simulink model "AllinOne"  (R2017a)
settings: Solver=ode3  StartTime=0.0  StopTime=Inf  RelTol=1e-3  EnableMultiTasking=on
StopFcn:
  | CoffeeMachineIOSupport('closefig');
libraries: pil_lib x1
settings Model: DataDictionary=Struct.sldd  NumberOfSteps=100  ParamWorkspaceSource=ReferencedWorkspace  Creator=89YY  LastModifiedBy=dell1
settings DataIOCC: LimitDataPoints=on  SaveFormat=Array
settings OptimizationCC: UseFloatMulNetSlope=on  PassReuseOutputArgsAs=Individual arguments  ZeroExternalMemoryAtStartup=off  ZeroInternalMemoryAtStartup=off  NoFixptDivByZeroProtection=on  EfficientFloat2IntCast=on  LifeSpan=1  MaxStackSize=64
settings DebuggingCC: SaveWithParameterizedLinksMsg=none  UnderspecifiedInitializationDetection=Classic  MergeDetectMultiDrivingBlocksExec=none  SFUnexpectedBacktrackingDiag=warning  SFNoUnconditionalDefaultTransitionDiag=warning  SFExecutionAtInitializationDiag=none
settings HardwareCC: ProdBitPerPointer=32  ProdBitPerSizeT=32  ProdBitPerPtrDiffT=32  ProdLargestAtomicInteger=Long  ProdLargestAtomicFloat=Double  ProdWordSize=32  ProdHWDeviceType=ARM Compatible->ARM Cortex  TargetBitPerPointer=64  TargetBitPerSizeT=64  TargetBitPerPtrDiffT=64  TargetLongLongMode=on  TargetIntDivRoundTo=Zero  TargetEndianess=LittleEndian  TargetWordSize=64  TargetHWDeviceType=MATLAB Host  ProdEqTarget=off
settings ModelReferenceCC: PropagateSignalLabelsOutOfModel=off
settings SFSimCC: MATLABDynamicMemAlloc=off
settings RTWCC: SystemTargetFile=ert.tlc  HardwareBoard=ARM Cortex-M3 (QEMU)  TLCOptions=-aInlineSetEventsForThisBaseRateFcn=TLC_FALSE -aSuppressMultiTaskScheduler=TLC_FALSE -aRateBasedStepFcn=1  TemplateMakefile=ert_default_tmf  Description=Embedded Coder  GenerateReport=on  Toolchain=GNU Tools for ARM Embedded Processors  IncludeHyperlinkInReport=on  LaunchReport=on  CreateSILPILBlock=PIL  GenerateTraceInfo=on  GenerateTraceReport=on  GenerateTraceReportSl=on  GenerateTraceReportSf=on  GenerateTraceReportEml=on  GenerateCodeMetricsReport=on
settings CodeAppCC: ForceParamTrailComments=on  IgnoreCustomStorageClasses=off  SimulinkDataObjDesc=on  CustomSymbolStrGlobalVar=rt$N$M  CustomSymbolStrType=$N$M  CustomSymbolStrFcn=$N$M$F  CustomSymbolStrMacro=$N$M  InsertBlockDesc=on
settings ERTTargetCC: MultiwordLength=2048  IncludeMdlTerminateFcn=off  CombineSignalStateStructs=on  SupportNonFinite=off  ERTFilePackagingFormat=CompactWithDataFile  ConvertIfToSwitch=off  SuppressUnreachableDefaultCases=off
settings ConfigComp: CovMetricSettings=dw  CovHtmlReporting=on  CovSaveCumulativeToWorkspaceVar=on  CovSaveSingleToWorkspaceVar=on  CovExternalEMLEnable=off  CovSFcnEnable=off

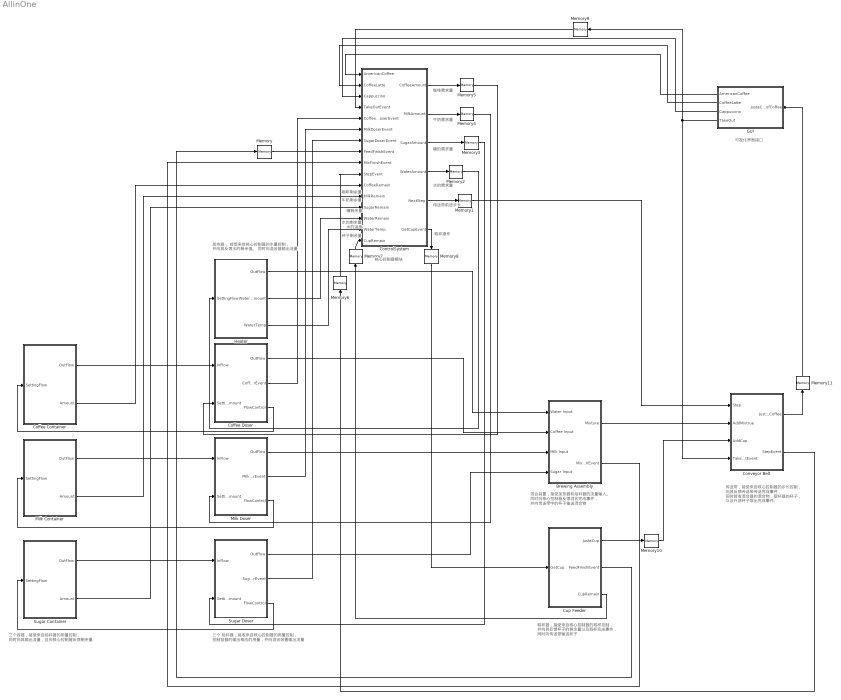
== system AllinOne ==
  note: 水的需求量
  note: 可视化界面接口
  note: 加热器， 接受来自核心控制器的水量控制，
      | 并向其反馈水的剩余值。
      | 同时向混合器输出流量
  note: 传送带，接受来自核心控制器的步长控制，
      | 向其反馈传送带传送完成事件，
      | 同时接收混合器的混合物，取杯器的杯子，
      | 以及外部杯子取出完成事件。
  note: 混合装置，接受加热器和给料器的流量输入。
      | 同时向核心控制器反馈混合完成事件，
      | 并向传送带中的杯子输送混合物
  note: 取杯器，接受来自核心控制器的取杯控制，
      | 并向其反馈杯子的剩余量以及取杯完成事件，
      | 同时向传送带输送杯子
  note: 三个 给料器，接收来自核心控制器的用量控制，
      | 控制容器的输出相应的用量，并向混合装置输出流量
  note: 三个容器，接受来自给料器的用量控制，
      | 同时向其输出流量，且向核心控制器反馈剩余量
  note: 取杯操作
  note: 传送带前进步长
  note: 糖的需求量
  note: 牛奶需求量
  note: 咖啡需求量
  note: 杯子剩余量
  note: 水的温度
  note: 水的剩余量
  note: 糖剩余量
  note: 牛奶剩余量
  note: 咖啡剩余量
  note: 核心控制器模块
  Brewing Assembly : Subsystem
  Coffee Container : Subsystem
  Coffee Doser : Subsystem
  ControlSystem : Subsystem  DialogController=pil_create_dialog  LoadFcn=|
      | try
      |    if ~strcmp(rtw.pil.getPILVersion, '6.12 (R2017a)_12')
      |       set_param(gcb, 'DialogController', '');
      |       set_param(gcb, 'DialogControllerArgs', '');
      |    end
      | catch e
      |       set_param(gcb, 'DialogController', '');
      |       set_param(gcb, 'DialogControllerArgs', '');
      | end
      mask help: PIL:pil:XILBlockMaskDesc
      mask Display: disp('PIL');
  Conveyor Belt : Subsystem
  Cup Feeder : Subsystem
  GUI : Subsystem
  Heater : Subsystem
  Memory{,1..11} (12 alike) : Memory
  Milk Container : Subsystem
  Milk Doser : Subsystem
  Sugar Container : Subsystem
  Sugar Doser : Subsystem
  wires:
  Milk Container/1(OutFlow) -> Milk Doser/1(InFlow)
  Milk Doser/3(FlowControl) -> Milk Container/1(SettingFlow)
  Coffee Container/1(OutFlow) -> Coffee Doser/1(InFlow)
  Coffee Doser/3(FlowControl) -> Coffee Container/1(SettingFlow)
  Sugar Container/1(OutFlow) -> Sugar Doser/1(InFlow)
  Sugar Doser/3(FlowControl) -> Sugar Container/1(SettingFlow)
  Coffee Doser/1(OutFlow) -> Brewing Assembly/2(Coffee Input)
  Milk Doser/1(OutFlow) -> Brewing Assembly/3(Milk Input)
  Sugar Doser/1(OutFlow) -> Brewing Assembly/4(Sugar Input)
  Brewing Assembly/1(Mixture) -> Conveyor Belt/2(AddMixtrue)
  Cup Feeder/1(JustaCup) -> Memory10/1
  Heater/1(OutFlow) -> Brewing Assembly/1(Water Input)
  GUI/4(TakeOut) -> Memory9/1, Conveyor Belt/4(TakeOutEvent)
  Conveyor Belt/1(JustaCupofCoffee) -> Memory11/1
  GUI/3(Cappuccino) -> ControlSystem/3(Cappuccino)
  GUI/2(CoffeeLatte) -> ControlSystem/2(CoffeeLatte)
  GUI/1(AmericanCoffee) -> ControlSystem/1(AmericanCoffee)
  Coffee Doser/2(CoffeeDoserEvent) -> ControlSystem/5(CoffeeDoserEvent)
  Milk Doser/2(MilkDoserEvent) -> ControlSystem/6(MilkDoserEvent)
  Sugar Doser/2(SugarDoserEvent) -> ControlSystem/7(SugarDoserEvent)
  Coffee Container/2(Amount) -> ControlSystem/11(CoffeeRemain)
  Milk Container/2(Amount) -> ControlSystem/12(MilkRemain)
  Sugar Container/2(Amount) -> ControlSystem/13(SugarRemain)
  Heater/2(WaterAmount) -> ControlSystem/14(WaterRemain)
  Heater/3(WaterTemp) -> ControlSystem/15(WaterTemp)
  Cup Feeder/3(CupRemain) -> Memory7/1
  Brewing Assembly/2(MixFinishEvent) -> ControlSystem/9(MixFinishEvent)
  Cup Feeder/2(FeedFinishEvent) -> Memory/1
  Conveyor Belt/2(StepEvent) -> Memory6/1
  ControlSystem/1(CoffeeAmount) -> Memory5/1
  ControlSystem/2(MilkAmount) -> Memory4/1
  ControlSystem/3(SugarAmount) -> Memory3/1
  ControlSystem/5(NextStep) -> Memory1/1
  ControlSystem/4(WaterAmount) -> Memory2/1
  Memory5/1 -> Coffee Doser/2(SettingAmount)
  Memory4/1 -> Milk Doser/2(SettingAmount)
  Memory3/1 -> Sugar Doser/2(SettingAmount)
  Memory2/1 -> Heater/1(SettingFlow)
  Memory1/1 -> Conveyor Belt/1(Step)
  ControlSystem/6(GetCupEvent) -> Memory8/1
  Memory/1 -> ControlSystem/8(FeedFinishEvent)
  Memory6/1 -> ControlSystem/10(StepEvent)
  Memory7/1 -> ControlSystem/16(CupRemain)
  Memory8/1 -> Cup Feeder/1(GetCup)
  Memory9/1 -> ControlSystem/4(TakeOutEvent)
  Memory10/1 -> Conveyor Belt/3(AddCup)
  Memory11/1 -> GUI/1(JustaCupofCoffee)

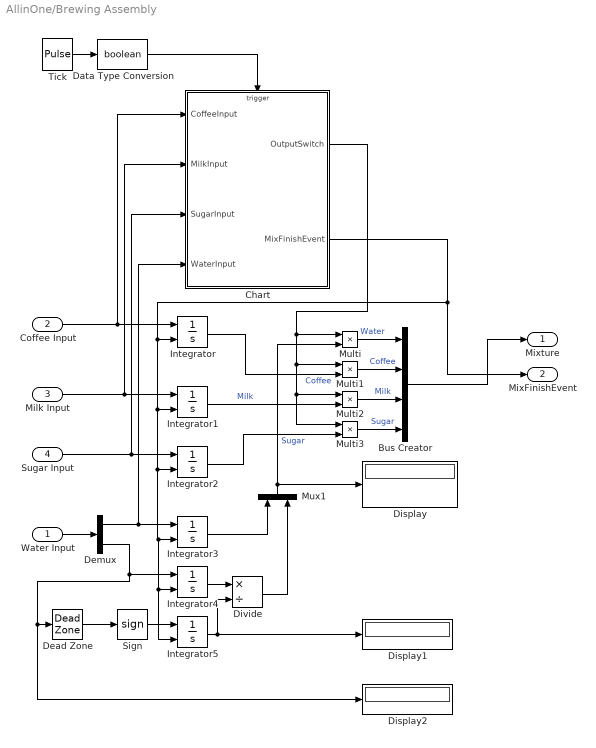
== system AllinOne/Brewing Assembly ==
  Water Input : Inport
  Coffee Input : Inport  Port=2
  Milk Input : Inport  Port=3
  Sugar Input : Inport  Port=4
  Bus Creator : BusCreator  Inputs=4  OutDataTypeStr=Bus: Mixtrue
  Chart : Stateflow chart  TreatAsAtomicUnit=on
  Data Type Conversion : DataTypeConversion  OutDataTypeStr=boolean
  Dead Zone : DeadZone  LowerValue=-1e-5  UpperValue=1e-5  SaturateOnIntegerOverflow=on
  Demux : Demux  Outputs=2
  Display : Display
  Display1 : Display
  Display2 : Display
  Divide : Product  Inputs=*/
  Integrator{,1..5} (6 alike) : Integrator  ExternalReset=rising
  Multi{,1..3} (4 alike) : Product  Inputs=**
  Mux1 : Mux  Inputs=2
  Sign : Signum
  Tick : DiscretePulseGenerator  PulseType=Time based  Period=0.01  PulseWidth=50
  Mixture : Outport  OutDataTypeStr=Bus: Mixtrue
  MixFinishEvent : Outport  Port=2
  wires:
  Tick/1 -> Data Type Conversion/1
  Data Type Conversion/1 -> Chart/Trigger
  Sugar Input/1 -> Integrator2/1, Chart/3(SugarInput)
  Demux/1 -> Chart/4(WaterInput), Integrator3/1
  Milk Input/1 -> Integrator1/1, Chart/2(MilkInput)
  Coffee Input/1 -> Integrator/1, Chart/1(CoffeeInput)
  Chart/2(MixFinishEvent) -> MixFinishEvent/1, Integrator5/2, Integrator4/2, Integrator3/2, Integrator2/2, Integrator1/2, Integrator/2
  Multi1/1 -> Bus Creator/2  "Coffee"
  Mux1/1 -> Multi/2, Display/1
  Multi2/1 -> Bus Creator/3  "Milk"
  Multi3/1 -> Bus Creator/4  "Sugar"
  Bus Creator/1 -> Mixture/1
  Chart/1(OutputSwitch) -> Multi3/1, Multi2/1, Multi1/1, Multi/1
  Water Input/1 -> Demux/1
  Integrator3/1 -> Mux1/1
  Sign/1 -> Integrator5/1
  Demux/2 -> Display2/1, Dead Zone/1, Integrator4/1
  Integrator4/1 -> Divide/1
  Integrator5/1 -> Display1/1, Divide/2
  Divide/1 -> Mux1/2
  Multi/1 -> Bus Creator/1  "Water"
  Integrator/1 -> Multi1/2  "Coffee"
  Integrator1/1 -> Multi2/2  "Milk"
  Integrator2/1 -> Multi3/2  "Sugar"
  Dead Zone/1 -> Sign/1

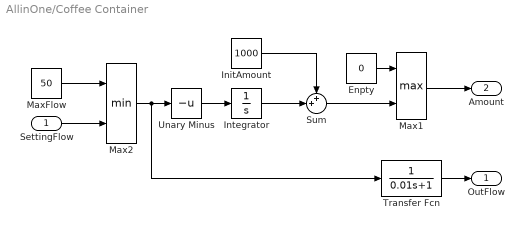
== system AllinOne/Coffee Container ==
  SettingFlow : Inport
  Enpty : Constant  Value=0
  InitAmount : Constant  Value=1000
  Integrator : Integrator
  Max1 : MinMax  Function=max  Inputs=2
  Max2 : MinMax  Inputs=2  OutMin=[0]
  MaxFlow : Constant  Value=50
  Sum : Sum  Inputs=++|
  Transfer Fcn : TransferFcn  Denominator=[0.01 1]
  Unary Minus : UnaryMinus
  OutFlow : Outport
  Amount : Outport  Port=2
  wires:
  Unary Minus/1 -> Integrator/1
  Integrator/1 -> Sum/2
  SettingFlow/1 -> Max2/2
  InitAmount/1 -> Sum/1
  Max2/1 -> Transfer Fcn/1, Unary Minus/1
  MaxFlow/1 -> Max2/1
  Max1/1 -> Amount/1
  Sum/1 -> Max1/2
  Enpty/1 -> Max1/1
  Transfer Fcn/1 -> OutFlow/1

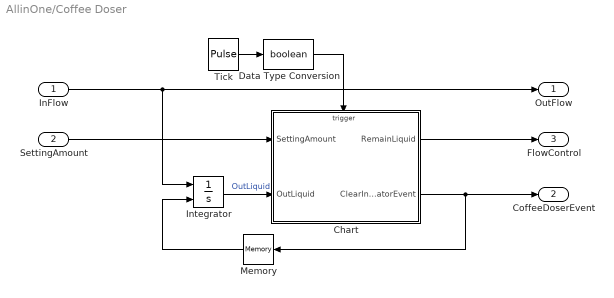
== system AllinOne/Coffee Doser ==
  InFlow : Inport
  SettingAmount : Inport  Port=2
  Chart : Stateflow chart  RequirementInfo={} %GIDa_ffed56c2_cd34_4288_8248_c4489554cc95  TreatAsAtomicUnit=on
  Data Type Conversion : DataTypeConversion  OutDataTypeStr=boolean
  Integrator : Integrator  ExternalReset=rising
  Memory : Memory
  Tick : DiscretePulseGenerator  PulseType=Time based  Period=0.01  PulseWidth=50
  OutFlow : Outport
  CoffeeDoserEvent : Outport  Port=2
  FlowControl : Outport  Port=3
  wires:
  SettingAmount/1 -> Chart/1(SettingAmount)
  Chart/1(RemainLiquid) -> FlowControl/1
  InFlow/1 -> OutFlow/1, Integrator/1
  Chart/2(ClearIntegratorEvent) -> Memory/1, CoffeeDoserEvent/1
  Integrator/1 -> Chart/2(OutLiquid)  "OutLiquid"
  Tick/1 -> Data Type Conversion/1
  Data Type Conversion/1 -> Chart/Trigger
  Memory/1 -> Integrator/2

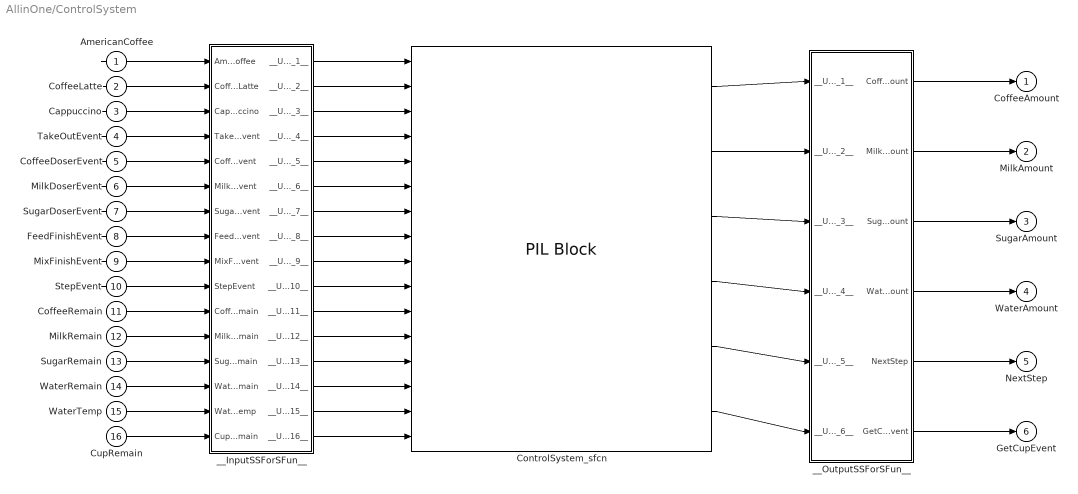
== system AllinOne/ControlSystem ==
  AmericanCoffee : Inport
  CoffeeLatte : Inport  Port=2
  Cappuccino : Inport  Port=3
  TakeOutEvent : Inport  Port=4
  CoffeeDoserEvent : Inport  Port=5
  MilkDoserEvent : Inport  Port=6
  SugarDoserEvent : Inport  Port=7
  FeedFinishEvent : Inport  Port=8
  MixFinishEvent : Inport  Port=9
  StepEvent : Inport  Port=10
  CoffeeRemain : Inport  Port=11
  MilkRemain : Inport  Port=12
  SugarRemain : Inport  Port=13
  WaterRemain : Inport  Port=14
  WaterTemp : Inport  Port=15
  CupRemain : Inport  Port=16
  ControlSystem_sfcn : pil_lib/PIL Block  SimulationMode=PIL  IsTopModelPIL=off  CodeDir=C:\Users\dell1\Desktop\coffee_machine\model\prepare\ControlSystem_ert_rtw  ConfigName=ARM Cortex-M3 (QEMU)  XrelIsTopModelCode=on
  __InputSSForSFun__ : Subsystem
  __OutputSSForSFun__ : Subsystem
  CoffeeAmount : Outport
  MilkAmount : Outport  Port=2
  SugarAmount : Outport  Port=3
  WaterAmount : Outport  Port=4
  NextStep : Outport  Port=5
  GetCupEvent : Outport  Port=6
  wires:
  __OutputSSForSFun__/6(GetCupEvent) -> GetCupEvent/1
  __OutputSSForSFun__/5(NextStep) -> NextStep/1
  __OutputSSForSFun__/4(WaterAmount) -> WaterAmount/1
  __OutputSSForSFun__/3(SugarAmount) -> SugarAmount/1
  __OutputSSForSFun__/2(MilkAmount) -> MilkAmount/1
  __OutputSSForSFun__/1(CoffeeAmount) -> CoffeeAmount/1
  ControlSystem_sfcn/6 -> __OutputSSForSFun__/6(__UniqueInportName__6__)
  ControlSystem_sfcn/5 -> __OutputSSForSFun__/5(__UniqueInportName__5__)
  ControlSystem_sfcn/4 -> __OutputSSForSFun__/4(__UniqueInportName__4__)
  ControlSystem_sfcn/3 -> __OutputSSForSFun__/3(__UniqueInportName__3__)
  ControlSystem_sfcn/2 -> __OutputSSForSFun__/2(__UniqueInportName__2__)
  ControlSystem_sfcn/1 -> __OutputSSForSFun__/1(__UniqueInportName__1__)
  __InputSSForSFun__/16(__UniqueOutportName__16__) -> ControlSystem_sfcn/16
  __InputSSForSFun__/15(__UniqueOutportName__15__) -> ControlSystem_sfcn/15
  __InputSSForSFun__/14(__UniqueOutportName__14__) -> ControlSystem_sfcn/14
  __InputSSForSFun__/13(__UniqueOutportName__13__) -> ControlSystem_sfcn/13
  __InputSSForSFun__/12(__UniqueOutportName__12__) -> ControlSystem_sfcn/12
  __InputSSForSFun__/11(__UniqueOutportName__11__) -> ControlSystem_sfcn/11
  __InputSSForSFun__/10(__UniqueOutportName__10__) -> ControlSystem_sfcn/10
  __InputSSForSFun__/9(__UniqueOutportName__9__) -> ControlSystem_sfcn/9
  __InputSSForSFun__/8(__UniqueOutportName__8__) -> ControlSystem_sfcn/8
  __InputSSForSFun__/7(__UniqueOutportName__7__) -> ControlSystem_sfcn/7
  __InputSSForSFun__/6(__UniqueOutportName__6__) -> ControlSystem_sfcn/6
  __InputSSForSFun__/5(__UniqueOutportName__5__) -> ControlSystem_sfcn/5
  __InputSSForSFun__/4(__UniqueOutportName__4__) -> ControlSystem_sfcn/4
  __InputSSForSFun__/3(__UniqueOutportName__3__) -> ControlSystem_sfcn/3
  __InputSSForSFun__/2(__UniqueOutportName__2__) -> ControlSystem_sfcn/2
  __InputSSForSFun__/1(__UniqueOutportName__1__) -> ControlSystem_sfcn/1
  CupRemain/1 -> __InputSSForSFun__/16(CupRemain)
  WaterTemp/1 -> __InputSSForSFun__/15(WaterTemp)
  WaterRemain/1 -> __InputSSForSFun__/14(WaterRemain)
  SugarRemain/1 -> __InputSSForSFun__/13(SugarRemain)
  MilkRemain/1 -> __InputSSForSFun__/12(MilkRemain)
  CoffeeRemain/1 -> __InputSSForSFun__/11(CoffeeRemain)
  StepEvent/1 -> __InputSSForSFun__/10(StepEvent)
  MixFinishEvent/1 -> __InputSSForSFun__/9(MixFinishEvent)
  FeedFinishEvent/1 -> __InputSSForSFun__/8(FeedFinishEvent)
  SugarDoserEvent/1 -> __InputSSForSFun__/7(SugarDoserEvent)
  MilkDoserEvent/1 -> __InputSSForSFun__/6(MilkDoserEvent)
  CoffeeDoserEvent/1 -> __InputSSForSFun__/5(CoffeeDoserEvent)
  TakeOutEvent/1 -> __InputSSForSFun__/4(TakeOutEvent)
  Cappuccino/1 -> __InputSSForSFun__/3(Cappuccino)
  CoffeeLatte/1 -> __InputSSForSFun__/2(CoffeeLatte)
  AmericanCoffee/1 -> __InputSSForSFun__/1(AmericanCoffee)

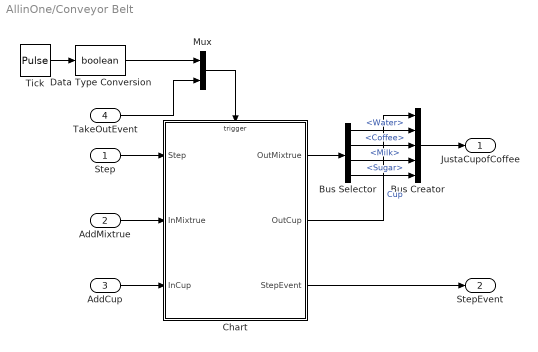
== system AllinOne/Conveyor Belt ==
  Step : Inport
  AddMixtrue : Inport  Port=2
  AddCup : Inport  Port=3
  TakeOutEvent : Inport  Port=4
  Bus Creator : BusCreator  Inputs=5
  Bus Selector : BusSelector  OutputSignals=Water,Coffee,Milk,Sugar
  Chart : Stateflow chart  TreatAsAtomicUnit=on
  Data Type Conversion : DataTypeConversion  OutDataTypeStr=boolean
  Mux : Mux  Inputs=2
  Tick : DiscretePulseGenerator  PulseType=Time based  Period=0.01  PulseWidth=50
  JustaCupofCoffee : Outport  OutDataTypeStr=Bus: aCupofCoffee
  StepEvent : Outport  Port=2
  wires:
  Tick/1 -> Data Type Conversion/1
  Data Type Conversion/1 -> Mux/1
  Chart/3(StepEvent) -> StepEvent/1
  AddCup/1 -> Chart/3(InCup)
  AddMixtrue/1 -> Chart/2(InMixtrue)
  Step/1 -> Chart/1(Step)
  Chart/1(OutMixtrue) -> Bus Selector/1
  Bus Selector/1 -> Bus Creator/2  "<Water>"
  Bus Selector/2 -> Bus Creator/3  "<Coffee>"
  Bus Selector/3 -> Bus Creator/4  "<Milk>"
  Bus Selector/4 -> Bus Creator/5  "<Sugar>"
  Chart/2(OutCup) -> Bus Creator/1  "Cup"
  Bus Creator/1 -> JustaCupofCoffee/1
  Mux/1 -> Chart/Trigger
  TakeOutEvent/1 -> Mux/2

== system AllinOne/Cup Feeder ==
  GetCup : Inport
  Chart : Stateflow chart  TreatAsAtomicUnit=on
  Data Type Conversion : DataTypeConversion  OutDataTypeStr=boolean
  Mux : Mux  Inputs=2
  Tick : DiscretePulseGenerator  PulseType=Time based  Period=0.01  PulseWidth=50
  JustaCup : Outport
  FeedFinishEvent : Outport  Port=2
  CupRemain : Outport  Port=3
  wires:
  Chart/1(JustaCup) -> JustaCup/1
  Chart/2(CupRemain) -> CupRemain/1
  Chart/3(FeedFinishEvent) -> FeedFinishEvent/1
  GetCup/1 -> Mux/2
  Tick/1 -> Data Type Conversion/1
  Mux/1 -> Chart/Trigger
  Data Type Conversion/1 -> Mux/1

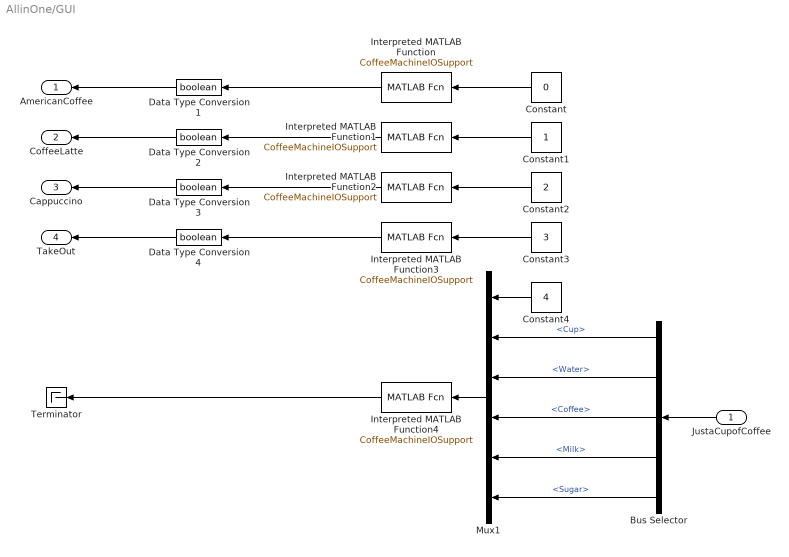
== system AllinOne/GUI ==
  JustaCupofCoffee : Inport
  Bus Selector : BusSelector  OutputSignals=Cup,Water,Coffee,Milk,Sugar
  Constant : Constant  Value=0
  Constant1 : Constant
  Constant2 : Constant  Value=2
  Constant3 : Constant  Value=3
  Constant4 : Constant  Value=4
  Data Type Conversion{1..4} (4 alike) : DataTypeConversion  OutDataTypeStr=boolean
  Interpreted MATLAB Function{,1..4} (5 alike) : MATLABFcn  MATLABFcn=CoffeeMachineIOSupport
  Mux1 : Mux  Inputs=6
  Terminator : Terminator
  AmericanCoffee : Outport
  CoffeeLatte : Outport  Port=2
  Cappuccino : Outport  Port=3
  TakeOut : Outport  Port=4
  wires:
  JustaCupofCoffee/1 -> Bus Selector/1
  Interpreted MATLAB Function3/1 -> Data Type Conversion4/1
  Interpreted MATLAB Function2/1 -> Data Type Conversion3/1
  Mux1/1 -> Interpreted MATLAB Function4/1
  Bus Selector/1 -> Mux1/2  "<Cup>"
  Bus Selector/3 -> Mux1/4  "<Coffee>"
  Bus Selector/4 -> Mux1/5  "<Milk>"
  Bus Selector/5 -> Mux1/6  "<Sugar>"
  Constant/1 -> Interpreted MATLAB Function/1
  Constant1/1 -> Interpreted MATLAB Function1/1
  Interpreted MATLAB Function/1 -> Data Type Conversion1/1
  Bus Selector/2 -> Mux1/3  "<Water>"
  Interpreted MATLAB Function1/1 -> Data Type Conversion2/1
  Constant4/1 -> Mux1/1
  Constant2/1 -> Interpreted MATLAB Function2/1
  Constant3/1 -> Interpreted MATLAB Function3/1
  Interpreted MATLAB Function4/1 -> Terminator/1
  Data Type Conversion2/1 -> CoffeeLatte/1
  Data Type Conversion1/1 -> AmericanCoffee/1
  Data Type Conversion3/1 -> Cappuccino/1
  Data Type Conversion4/1 -> TakeOut/1

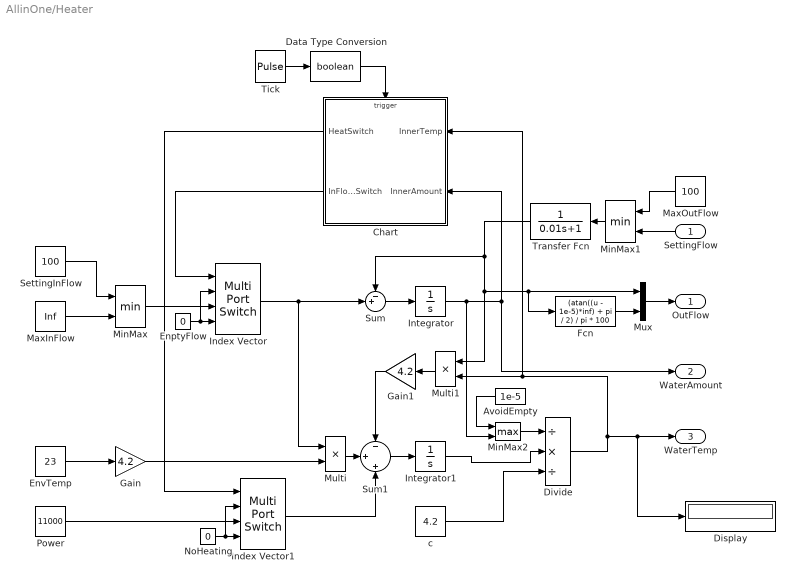
== system AllinOne/Heater ==
  SettingFlow : Inport
  AvoidEmpty : Constant  Value=1e-5
  Chart : Stateflow chart  TreatAsAtomicUnit=on
  Data Type Conversion : DataTypeConversion  OutDataTypeStr=boolean
  Display : Display
  Divide : Product  Inputs=/*/
  EnptyFlow : Constant  Value=0
  EnvTemp : Constant  Value=23
  Fcn : Fcn  Expr=(atan((u - 1e-5)*inf) + pi / 2) / pi * 100
  Gain : Gain  Gain=4.2
  Gain1 : Gain  Gain=4.2
  Index Vector : MultiPortSwitch  DataPortOrder=Zero-based contiguous  Inputs=2  DataPortForDefault=Additional data port  DiagnosticForDefault=None  zeroidx=on
  Index Vector1 : MultiPortSwitch  DataPortOrder=Zero-based contiguous  Inputs=2  DataPortForDefault=Additional data port  DiagnosticForDefault=None  zeroidx=on
  Integrator : Integrator
  Integrator1 : Integrator
  MaxInFlow : Constant  Value=Inf
  MaxOutFlow : Constant  Value=100
  MinMax : MinMax  Inputs=2
  MinMax1 : MinMax  Inputs=2
  MinMax2 : MinMax  Function=max  Inputs=2
  Multi : Product  Inputs=**
  Multi1 : Product  Inputs=**
  Mux : Mux  Inputs=2
  NoHeating : Constant  Value=0
  Power : Constant  Value=11000
  SettingInFlow : Constant  Value=100
  Sum : Sum  Inputs=-+|
  Sum1 : Sum  Inputs=-|+|+
  Tick : DiscretePulseGenerator  PulseType=Time based  Period=0.01  PulseWidth=50
  Transfer Fcn : TransferFcn  Denominator=[0.01 1]
  c : Constant  Value=4.2
  OutFlow : Outport
  WaterAmount : Outport  Port=2
  WaterTemp : Outport  Port=3
  wires:
  MaxInFlow/1 -> MinMax/2
  SettingInFlow/1 -> MinMax/1
  Sum/1 -> Integrator/1
  Sum1/1 -> Integrator1/1
  EnvTemp/1 -> Gain/1
  Integrator/1 -> MinMax2/2, WaterAmount/1, Chart/2(InnerAmount)
  Integrator1/1 -> Divide/2
  c/1 -> Divide/3
  Gain/1 -> Multi/2
  Multi/1 -> Sum1/2
  Index Vector/1 -> Multi/1, Sum/2
  EnptyFlow/1 -> Index Vector/2, Index Vector/4
  MinMax/1 -> Index Vector/3
  Chart/2(InFlowSwitch) -> Index Vector/1
  NoHeating/1 -> Index Vector1/2, Index Vector1/4
  Chart/1(HeatSwitch) -> Index Vector1/1
  Index Vector1/1 -> Sum1/3
  Power/1 -> Index Vector1/3
  MaxOutFlow/1 -> MinMax1/1
  SettingFlow/1 -> MinMax1/2
  MinMax1/1 -> Transfer Fcn/1
  Mux/1 -> OutFlow/1
  Transfer Fcn/1 -> Fcn/1, Mux/1, Multi1/1, Sum/1
  Tick/1 -> Data Type Conversion/1
  Data Type Conversion/1 -> Chart/Trigger
  Multi1/1 -> Gain1/1
  Gain1/1 -> Sum1/1
  MinMax2/1 -> Divide/1
  AvoidEmpty/1 -> MinMax2/1
  Divide/1 -> Multi1/2, Chart/1(InnerTemp), Display/1, WaterTemp/1
  Fcn/1 -> Mux/2

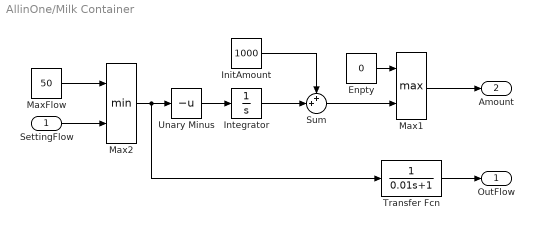
== system AllinOne/Milk Container ==
  SettingFlow : Inport
  Enpty : Constant  Value=0
  InitAmount : Constant  Value=1000
  Integrator : Integrator
  Max1 : MinMax  Function=max  Inputs=2
  Max2 : MinMax  Inputs=2  OutMin=[0]
  MaxFlow : Constant  Value=50
  Sum : Sum  Inputs=++|
  Transfer Fcn : TransferFcn  Denominator=[0.01 1]
  Unary Minus : UnaryMinus
  OutFlow : Outport
  Amount : Outport  Port=2
  wires:
  Unary Minus/1 -> Integrator/1
  Integrator/1 -> Sum/2
  SettingFlow/1 -> Max2/2
  InitAmount/1 -> Sum/1
  Max2/1 -> Transfer Fcn/1, Unary Minus/1
  MaxFlow/1 -> Max2/1
  Max1/1 -> Amount/1
  Sum/1 -> Max1/2
  Enpty/1 -> Max1/1
  Transfer Fcn/1 -> OutFlow/1

== system AllinOne/Milk Doser ==
  InFlow : Inport
  SettingAmount : Inport  Port=2
  Chart : Stateflow chart  RequirementInfo={} %GIDa_551bb34e_10e7_4a73_950c_ffc9537d9666  TreatAsAtomicUnit=on
  Data Type Conversion : DataTypeConversion  OutDataTypeStr=boolean
  Integrator : Integrator  ExternalReset=rising
  Memory : Memory
  Tick : DiscretePulseGenerator  PulseType=Time based  Period=0.01  PulseWidth=50
  OutFlow : Outport
  MilkDoserEvent : Outport  Port=2
  FlowControl : Outport  Port=3
  wires:
  SettingAmount/1 -> Chart/1(SettingAmount)
  Chart/1(RemainLiquid) -> FlowControl/1
  InFlow/1 -> OutFlow/1, Integrator/1
  Chart/2(ClearIntegratorEvent) -> Memory/1, MilkDoserEvent/1
  Integrator/1 -> Chart/2(OutLiquid)  "OutLiquid"
  Tick/1 -> Data Type Conversion/1
  Data Type Conversion/1 -> Chart/Trigger
  Memory/1 -> Integrator/2

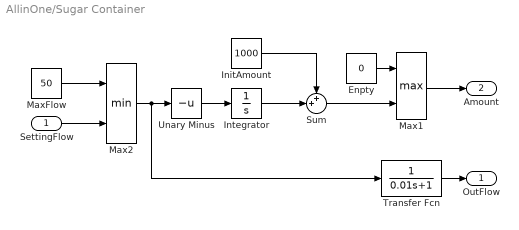
== system AllinOne/Sugar Container ==
  SettingFlow : Inport
  Enpty : Constant  Value=0
  InitAmount : Constant  Value=1000
  Integrator : Integrator
  Max1 : MinMax  Function=max  Inputs=2
  Max2 : MinMax  Inputs=2  OutMin=[0]
  MaxFlow : Constant  Value=50
  Sum : Sum  Inputs=++|
  Transfer Fcn : TransferFcn  Denominator=[0.01 1]
  Unary Minus : UnaryMinus
  OutFlow : Outport
  Amount : Outport  Port=2
  wires:
  Unary Minus/1 -> Integrator/1
  Integrator/1 -> Sum/2
  SettingFlow/1 -> Max2/2
  InitAmount/1 -> Sum/1
  Max2/1 -> Transfer Fcn/1, Unary Minus/1
  MaxFlow/1 -> Max2/1
  Max1/1 -> Amount/1
  Sum/1 -> Max1/2
  Enpty/1 -> Max1/1
  Transfer Fcn/1 -> OutFlow/1

== system AllinOne/Sugar Doser ==
  InFlow : Inport
  SettingAmount : Inport  Port=2
  Chart : Stateflow chart  RequirementInfo={} %GIDa_3f65ce12_bb97_4ef2_8d1d_79df95e5fb82  TreatAsAtomicUnit=on
  Data Type Conversion : DataTypeConversion  OutDataTypeStr=boolean
  Integrator : Integrator  ExternalReset=rising
  Memory : Memory
  Tick : DiscretePulseGenerator  PulseType=Time based  Period=0.01  PulseWidth=50
  OutFlow : Outport
  SugarDoserEvent : Outport  Port=2
  FlowControl : Outport  Port=3
  wires:
  SettingAmount/1 -> Chart/1(SettingAmount)
  Chart/1(RemainLiquid) -> FlowControl/1
  InFlow/1 -> OutFlow/1, Integrator/1
  Chart/2(ClearIntegratorEvent) -> Memory/1, SugarDoserEvent/1
  Integrator/1 -> Chart/2(OutLiquid)  "OutLiquid"
  Tick/1 -> Data Type Conversion/1
  Data Type Conversion/1 -> Chart/Trigger
  Memory/1 -> Integrator/2

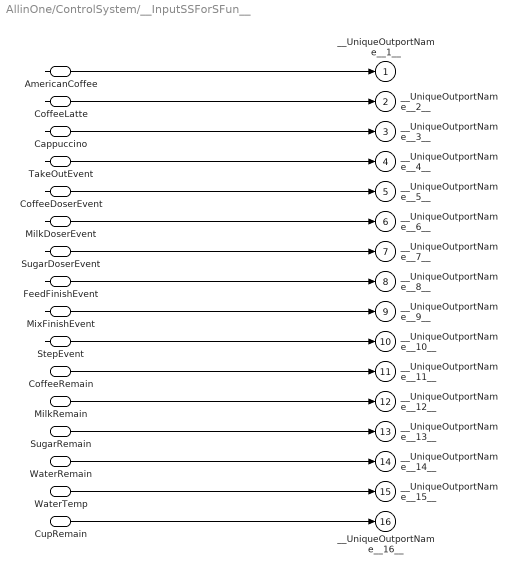
== system AllinOne/ControlSystem/__InputSSForSFun__ ==
  AmericanCoffee : Inport
  CoffeeLatte : Inport  Port=2
  Cappuccino : Inport  Port=3
  TakeOutEvent : Inport  Port=4
  CoffeeDoserEvent : Inport  Port=5
  MilkDoserEvent : Inport  Port=6
  SugarDoserEvent : Inport  Port=7
  FeedFinishEvent : Inport  Port=8
  MixFinishEvent : Inport  Port=9
  StepEvent : Inport  Port=10
  CoffeeRemain : Inport  Port=11
  MilkRemain : Inport  Port=12
  SugarRemain : Inport  Port=13
  WaterRemain : Inport  Port=14
  WaterTemp : Inport  Port=15
  CupRemain : Inport  Port=16
  __UniqueOutportName__1__ : Outport
  __UniqueOutportName__2__ : Outport  Port=2
  __UniqueOutportName__3__ : Outport  Port=3
  __UniqueOutportName__4__ : Outport  Port=4
  __UniqueOutportName__5__ : Outport  Port=5
  __UniqueOutportName__6__ : Outport  Port=6
  __UniqueOutportName__7__ : Outport  Port=7
  __UniqueOutportName__8__ : Outport  Port=8
  __UniqueOutportName__9__ : Outport  Port=9
  __UniqueOutportName__10__ : Outport  Port=10
  __UniqueOutportName__11__ : Outport  Port=11
  __UniqueOutportName__12__ : Outport  Port=12
  __UniqueOutportName__13__ : Outport  Port=13
  __UniqueOutportName__14__ : Outport  Port=14
  __UniqueOutportName__15__ : Outport  Port=15
  __UniqueOutportName__16__ : Outport  Port=16
  wires:
  CupRemain/1 -> __UniqueOutportName__16__/1
  WaterTemp/1 -> __UniqueOutportName__15__/1
  WaterRemain/1 -> __UniqueOutportName__14__/1
  SugarRemain/1 -> __UniqueOutportName__13__/1
  MilkRemain/1 -> __UniqueOutportName__12__/1
  CoffeeRemain/1 -> __UniqueOutportName__11__/1
  StepEvent/1 -> __UniqueOutportName__10__/1
  MixFinishEvent/1 -> __UniqueOutportName__9__/1
  FeedFinishEvent/1 -> __UniqueOutportName__8__/1
  SugarDoserEvent/1 -> __UniqueOutportName__7__/1
  MilkDoserEvent/1 -> __UniqueOutportName__6__/1
  CoffeeDoserEvent/1 -> __UniqueOutportName__5__/1
  TakeOutEvent/1 -> __UniqueOutportName__4__/1
  Cappuccino/1 -> __UniqueOutportName__3__/1
  CoffeeLatte/1 -> __UniqueOutportName__2__/1
  AmericanCoffee/1 -> __UniqueOutportName__1__/1

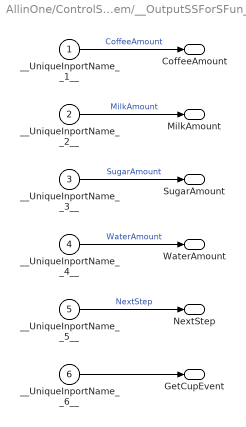
== system AllinOne/ControlSystem/__OutputSSForSFun__ ==
  __UniqueInportName__1__ : Inport
  __UniqueInportName__2__ : Inport  Port=2
  __UniqueInportName__3__ : Inport  Port=3
  __UniqueInportName__4__ : Inport  Port=4
  __UniqueInportName__5__ : Inport  Port=5
  __UniqueInportName__6__ : Inport  Port=6
  CoffeeAmount : Outport
  MilkAmount : Outport  Port=2
  SugarAmount : Outport  Port=3
  WaterAmount : Outport  Port=4
  NextStep : Outport  Port=5
  GetCupEvent : Outport  Port=6
  wires:
  __UniqueInportName__6__/1 -> GetCupEvent/1
  __UniqueInportName__5__/1 -> NextStep/1  "NextStep"
  __UniqueInportName__4__/1 -> WaterAmount/1  "WaterAmount"
  __UniqueInportName__3__/1 -> SugarAmount/1  "SugarAmount"
  __UniqueInportName__2__/1 -> MilkAmount/1  "MilkAmount"
  __UniqueInportName__1__/1 -> CoffeeAmount/1  "CoffeeAmount"

== stateflow chart AllinOne/Conveyor Belt/Chart ==
  settings: executeAtInitialization=1  initializeOutput=1
  state MixtrueMonitor [parallel]
    settings: executionOrder=2
    state Waiting
    state Adding
      en:
      LocalMixtrue = InMixtrue;
    MixtrueMonitor.Waiting -> MixtrueMonitor.Adding : [InMixtrue.Coffee > eps && ...
        | abs(CupLocation - 50) < 5]
    (default) -> MixtrueMonitor.Waiting
    MixtrueMonitor.Adding -> MixtrueMonitor.Waiting : [InMixtrue.Coffee <= eps]
  state CupMonitor [parallel]
    settings: executionOrder=3
    state Waiting
    state Adding
      en:
      CupLocation = 0;
    CupMonitor.Waiting -> CupMonitor.Adding : [InCup > eps && ...
        | CupLocation < 0]
    (default) -> CupMonitor.Waiting
    CupMonitor.Adding -> CupMonitor.Waiting : [InCup <=eps]
  state CupTransmit [parallel]
    settings: executionOrder=1
    state Start
      en:CupLocation = -1;
    state Running
    state Output
      du:
      OutMixtrue = LocalMixtrue;
      OutCup = 1;
      ex:
      OutMixtrue.Water = [0,0]';
      OutMixtrue.Coffee = 0;
      OutMixtrue.Milk = 0;
      OutMixtrue.Sugar = 0;
      OutCup = 0;
    state Prepare
    state Finished
    state Stepping
      en:
      CupLocation = CupLocation + Step;
      StepEvent;
      ex:
      StepEvent;
    Output -> Start : TakeOutEvent
    Start -> Running : [CupLocation >= 0]
    (default) -> Start
    Running -> Output [order 1] : [CupLocation >= 100]
    Finished -> Running : [Step < eps]
    Running -> Prepare [order 2] : [Step > eps && CupLocation >= 0]
    Prepare -> Stepping : [after(Step, Tick)]
    Stepping -> Finished : after(10, Tick)
  data: Step input; CupLocation local; InMixtrue input Bus: Mixtrue; OutMixtrue output Bus: Mixtrue; InCup input; OutCup output; LocalMixtrue local Bus: Mixtrue
  events: Tick input RISING_EDGE_EVENT; StepEvent output EITHER_EDGE_EVENT; TakeOutEvent input RISING_EDGE_EVENT

== stateflow chart AllinOne/Milk Doser/Chart ==
  settings: sampleTime=TIMER  executeAtInitialization=1
  state Ready
  state Finish
  state Transmiting
    entry: TargetAmount = SettingAmount; RemainLiquid = TargetAmount / 3;
    exit: RemainLiquid = 0;
  (default) -> Ready
  Finish -> Ready : [after(5, Tick) && SettingAmount==0]
      | {
      | 	send(ClearIntegratorEvent);
      | }
  Ready -> Transmiting : [SettingAmount > 0]
  Transmiting -> Finish : [TargetAmount - OutLiquid <= 0]
      | {
      | 	send(ClearIntegratorEvent);
      | }
  data: SettingAmount input; RemainLiquid output; OutLiquid input; TargetAmount local
  events: ClearIntegratorEvent output EITHER_EDGE_EVENT; Tick input RISING_EDGE_EVENT

== stateflow chart AllinOne/Sugar Doser/Chart ==
  settings: sampleTime=TIMER  executeAtInitialization=1
  state Ready
  state Finish
  state Transmiting
    entry: TargetAmount = SettingAmount; RemainLiquid = TargetAmount / 3;
    exit: RemainLiquid = 0;
  (default) -> Ready
  Finish -> Ready : [after(5, Tick) && SettingAmount==0]
      | {
      | 	send(ClearIntegratorEvent);
      | }
  Ready -> Transmiting : [SettingAmount > 0]
  Transmiting -> Finish : [TargetAmount - OutLiquid <= 0]
      | {
      | 	send(ClearIntegratorEvent);
      | }
  data: SettingAmount input; RemainLiquid output; OutLiquid input; TargetAmount local
  events: ClearIntegratorEvent output EITHER_EDGE_EVENT; Tick input RISING_EDGE_EVENT

== stateflow chart AllinOne/Coffee Doser/Chart ==
  settings: sampleTime=TIMER  executeAtInitialization=1
  state Ready
  state Finish
  state Transmiting
    entry: TargetAmount = SettingAmount; RemainLiquid = TargetAmount / 3;
    exit: RemainLiquid = 0;
  (default) -> Ready
  Finish -> Ready : [after(5, Tick) && SettingAmount==0]
      | {
      | 	send(ClearIntegratorEvent);
      | }
  Ready -> Transmiting : [SettingAmount > 0]
  Transmiting -> Finish : [TargetAmount - OutLiquid <= 0]
      | {
      | 	send(ClearIntegratorEvent);
      | }
  data: SettingAmount input; RemainLiquid output; OutLiquid input; TargetAmount local
  events: ClearIntegratorEvent output EITHER_EDGE_EVENT; Tick input RISING_EDGE_EVENT

== stateflow chart AllinOne/Cup Feeder/Chart ==
  settings: executeAtInitialization=1  initializeOutput=1
  state Ready
    du:
    CupRemain=[CupAmount>0;];
  state PutaCup
    entry:
    send(FeedFinishEvent);
    JustaCup = 1;
    CupAmount = CupAmount - 1;
    exit:
    JustaCup = 0;
    send(FeedFinishEvent);
  (default) -> Ready : {
      | 	CupAmount = 10;
      | 	JustaCup = 0;
      | }
  PutaCup -> Ready : after(5, Tick)
  Ready -> PutaCup : NeedCupEvent
  data: JustaCup output; CupRemain output; CupAmount local
  events: FeedFinishEvent output EITHER_EDGE_EVENT; Tick input RISING_EDGE_EVENT; NeedCupEvent input RISING_EDGE_EVENT

== stateflow chart AllinOne/Heater/Chart ==
  state InFlow [parallel]
    settings: executionOrder=2
    state GetInFlow
      en: InFlowSwitch = 1;
    state OFF
      en: InFlowSwitch = 0;
    GetInFlow -> InFlow.OFF : [InnerAmount>2000]
    (default) -> InFlow.OFF
    InFlow.OFF -> GetInFlow : [InnerAmount<1900]
  state Heater [parallel]
    settings: executionOrder=1
    state Heating
      en: HeatSwitch = 1;
    state OFF
      en: HeatSwitch = 0;
    Heating -> Heater.OFF : [InnerTemp>95]
    (default) -> Heater.OFF
    Heater.OFF -> Heating : [InnerTemp<80]
  data: InnerTemp input; InnerAmount input; HeatSwitch output; InFlowSwitch output
  events: Tick input RISING_EDGE_EVENT

== stateflow chart AllinOne/Brewing Assembly/Chart ==
  settings: executeAtInitialization=1  initializeOutput=1
  state WaterState [parallel]
    settings: executionOrder=1
    state Waiting
    state Adding
    state Finished
    (default) -> WaterState.Waiting
    WaterState.Finished -> WaterState.Waiting : LocalFinishEvent
    WaterState.Waiting -> WaterState.Adding : [WaterInput > 1e-5]
    WaterState.Adding -> WaterState.Finished : [WaterInput < 1e-5]
  state CoffeeState [parallel]
    settings: executionOrder=2
    state Waiting
    state Adding
    state Finished
    (default) -> CoffeeState.Waiting
    CoffeeState.Finished -> CoffeeState.Waiting : LocalFinishEvent
    CoffeeState.Waiting -> CoffeeState.Adding : [CoffeeInput > 1e-5]
    CoffeeState.Adding -> CoffeeState.Finished : [CoffeeInput < 1e-5]
  state MilkState [parallel]
    settings: executionOrder=3
    state Waiting
    state Adding
    state Finished
    (default) -> MilkState.Waiting
    MilkState.Finished -> MilkState.Waiting : LocalFinishEvent
    MilkState.Waiting -> MilkState.Adding : [MilkInput > 1e-5]
    MilkState.Adding -> MilkState.Finished : [MilkInput < 1e-5]
  state SugarState [parallel]
    settings: executionOrder=4
    state Waiting
    state Adding
    state Finished
    (default) -> SugarState.Waiting
    SugarState.Finished -> SugarState.Waiting : LocalFinishEvent
    SugarState.Waiting -> SugarState.Adding : [SugarInput > 1e-5]
    SugarState.Adding -> SugarState.Finished : [SugarInput < 1e-5]
  state Mix [parallel]
    settings: executionOrder=5
    state Waiting
    state Mixing
    state Output
      en:
      OutputSwitch = 1;
      ex:
      OutputSwitch = 0;
    state Finished
      en:
      MixFinishEvent;
      LocalFinishEvent;
    Mix.Waiting -> Mixing : [in(WaterState.Finished) && ...
        | in(CoffeeState.Finished) && ...
        | in(MilkState.Finished) && ...
        | in(SugarState.Finished)]
    Output -> Mix.Finished : after(5, Tick)
    Mixing -> Output : after(5, Tick)
    (default) -> Mix.Waiting : {OutputSwitch = 0;}
    Mix.Finished -> Mix.Waiting : [after(10,Tick) && ...
        | in(WaterState.Waiting) && ...
        | in(CoffeeState.Waiting) && ...
        | in(MilkState.Waiting) && ...
        | in(SugarState.Waiting)]/
        | {
        | 	MixFinishEvent;
        | 	LocalFinishEvent;
        | }
  data: CoffeeInput input; MilkInput input; SugarInput input; WaterInput input; OutputSwitch output
  events: Tick input RISING_EDGE_EVENT; MixFinishEvent output EITHER_EDGE_EVENT; LocalFinishEvent local FUNCTION_CALL_EVENT
